simulink model "starshotsimv5"  (R2021a)
settings: Solver=VariableStepAuto  StartTime=0.0  StopTime=6000  FixedStep=0.01  MaxStep=4.0  MinStep=.001  RelTol=1e-6
values from neighbouring files (symbols this model uses):
  B0 = 3.12e-5    (= 3.12e-05)    [starshot_ACS_setup.m]
  dT = 0.01    [scr_EKF.m]    (also in starshot_ACS_setup.m = 0.1)
  G = 6.67e-11    [starshot_ACS_setup.m]
  Hd = H    [scr_EKF.m]    (also in starshot_ACS_setup.m)
  k_noise = 1    [scr_EKF.m]    (also in starshot_ACS_setup.m = 3e-05)
  M_Earth = 5.972e24    (= 5.972e+24)    [starshot_ACS_setup.m]
  Q = [100,  0,  0 ... (first row only)    [scr_EKF.m]    (also in starshot_ACS_setup.m = 0.02*diag([0.008,0.07,0.005,0.1,0.1,0.1]))
  q0 = [qmatlab(2:4),qmatlab(1)]'    [starshot_ACS_setup.m]
  R_Earth = 6.378e6    (= 6378000)    [starshot_ACS_setup.m]
  Rd = (1/dT)*R    [scr_EKF.m]    (also in starshot_ACS_setup.m = Rn)
  Rn = [[ 2.02559220e-01,  5.17515015e-03, -3.16669361e-02, -1.76503506e-04, -3.74891174e-05, -7.75657503e-05] ... (first row only)    [starshot_ACS_setup.m]
undefined symbols (not defined in the file or in its folder): DiscIntNeverNeededParam, starshot
libraries: vrlib x2, simulink x2, dspmathops x1
settings Model: Creator=armen  LastModifiedBy=soumy
settings DataIOCC: SaveFormat=Array  ReturnWorkspaceOutputs=off
settings OptimizationCC: DefaultParameterBehavior=Inlined  UseDivisionForNetSlopeComputation=on  UseFloatMulNetSlope=on  InlineInvariantSignals=on  PassReuseOutputArgsAs=Individual arguments  ZeroExternalMemoryAtStartup=off  ZeroInternalMemoryAtStartup=off  NoFixptDivByZeroProtection=on  EfficientFloat2IntCast=on  LifeSpan=1  EfficientTunableParamExpr=on
settings DebuggingCC: ParameterTunabilityLossMsg=error  SFMachineParentedDataDiag=warning  ArithmeticOperatorsInVariantConditions=warning
settings HardwareCC: ProdBitPerPointer=32  ProdBitPerSizeT=32  ProdBitPerPtrDiffT=32  ProdLargestAtomicInteger=Long  ProdLargestAtomicFloat=Double  ProdWordSize=32  ProdHWDeviceType=ARM Compatible->ARM Cortex
settings SFSimCC: SimUseLocalCustomCode=off  MATLABDynamicMemAlloc=off  CustomCodeUndefinedFunction=UseInterfaceOnly  SimTargetLang=C++
settings RTWCC: SystemTargetFile=ert.tlc  GenCodeOnly=on  TemplateMakefile=ert_default_tmf  GenerateReport=on  RTWUseLocalCustomCode=off  IncludeHyperlinkInReport=on  LaunchReport=on  TargetLang=C++  GenerateTraceInfo=on  GenerateTraceReport=on  GenerateTraceReportSl=on  GenerateTraceReportSf=on  GenerateTraceReportEml=on
settings CodeAppCC: ForceParamTrailComments=on  IgnoreCustomStorageClasses=off  OperatorAnnotations=on  SimulinkDataObjDesc=on  SFDataObjDesc=on  MATLABFcnDesc=on  CustomSymbolStrGlobalVar=rt$N$M  CustomSymbolStrType=$N$M  CustomSymbolStrFcn=$N$M$F  CustomSymbolStrMacro=$N$M  InsertBlockDesc=on  StateflowObjectComments=on  MATLABSourceComments=on
settings ERTTargetCC: TargetLangStandard=C++03 (ISO)  GenerateSampleERTMain=on  IncludeMdlTerminateFcn=off  CombineSignalStateStructs=on  SupportAbsoluteTime=off  CodeInterfacePackaging=C++ class  SupportComplex=off  SupportNonInlinedSFcns=on  InlinedParameterPlacement=NonHierarchical  RootIOFormat=Structure reference  ERTCustomFileTemplate=example_file_process.tlc  ERTFilePackagingFormat=CompactWithDataFile

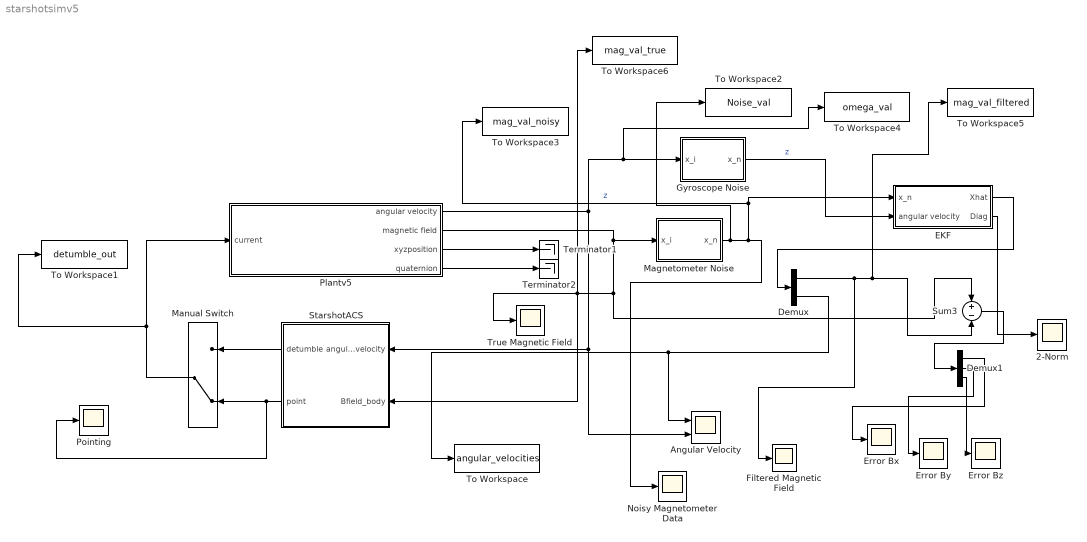
== system starshotsimv5 ==
  2-Norm : Scope
  Angular Velocity : Scope  NumInputPorts=2
  Demux : Demux  Outputs=2
  Demux1 : Demux  Outputs=3
  EKF : Subsystem  TreatAsAtomicUnit=on
      settings: MinAlgLoopOccurrences=on
  Error Bx : Scope
  Error By : Scope
  Error Bz : Scope
  Filtered Magnetic Field : Scope
  Gyroscope Noise : Subsystem
  Magnetometer Noise : Subsystem  TreatAsAtomicUnit=on
      settings: MinAlgLoopOccurrences=on
  Manual Switch : ManualSwitch  CurrentSetting=0
  Noisy Magnetometer Data : Scope
  Plantv5 : Subsystem  TreatAsAtomicUnit=on
  Pointing : Scope
  StarshotACS : Subsystem  TreatAsAtomicUnit=on
  Sum3 : Sum  Inputs=+-
  Terminator1 : Terminator
  Terminator2 : Terminator
  To Workspace : ToWorkspace  VariableName=angular_velocities  SaveFormat=Timeseries  SampleTime=-1
  To Workspace1 : ToWorkspace  VariableName=detumble_out  SaveFormat=Timeseries  SampleTime=-1
  To Workspace2 : ToWorkspace  VariableName=Noise_val  SaveFormat=Timeseries  SampleTime=-1
  To Workspace3 : ToWorkspace  VariableName=mag_val_noisy  SaveFormat=Timeseries  SampleTime=-1
  To Workspace4 : ToWorkspace  VariableName=omega_val  SaveFormat=Timeseries  SampleTime=-1
  To Workspace5 : ToWorkspace  VariableName=mag_val_filtered  SaveFormat=Timeseries  SampleTime=-1
  To Workspace6 : ToWorkspace  VariableName=mag_val_true  SaveFormat=Timeseries  SampleTime=-1
  True Magnetic Field : Scope
  wires:
  Plantv5/2(magnetic field) -> Sum3/1, StarshotACS/2(Bfield_body), To Workspace6/1, True Magnetic Field/1, Magnetometer Noise/1(x_i)
  Plantv5/1(angular velocity) -> To Workspace4/1, Gyroscope Noise/1(x_i), Angular Velocity/2, StarshotACS/1(angularvelocity)
  Plantv5/3(xyzposition) -> Terminator1/1
  Plantv5/4(quaternion) -> Terminator2/1
  StarshotACS/2(point) -> Pointing/1, Manual Switch/2
  StarshotACS/1(detumble) -> Manual Switch/1
  Manual Switch/1 -> To Workspace1/1, Plantv5/1(current)
  Magnetometer Noise/1(x_n) -> To Workspace2/1, To Workspace3/1, EKF/1(x_n), Noisy Magnetometer Data/1  "z"
  EKF/1(Xhat) -> Demux/1
  Demux/1 -> To Workspace5/1, Sum3/2, Filtered Magnetic Field/1
  Demux/2 -> To Workspace/1, Angular Velocity/1
  Gyroscope Noise/1(x_n) -> EKF/2(angular velocity)  "z"
  Sum3/1 -> Demux1/1
  Demux1/1 -> Error Bx/1
  Demux1/2 -> Error By/1
  Demux1/3 -> Error Bz/1
  EKF/2(Diag) -> 2-Norm/1

== system starshotsimv5/EKF ==
  x_n : Inport
  angular velocity : Inport  Port=2
  EKF_Primary : Subsystem
  Jacobian : MATLAB Function  TreatAsAtomicUnit=on
  Scope : Scope  NumInputPorts=2
  Vector Concatenate : Concatenate
  Xhat : Outport
  Diag : Outport  Port=2
  wires:
  EKF_Primary/2(sqrtPii) -> Diag/1
  Jacobian/1(J) -> EKF_Primary/2(J)
  EKF_Primary/1(Xhat) -> Scope/2, Xhat/1
  angular velocity/1 -> Vector Concatenate/2, Jacobian/2(angular_velocities)
  x_n/1 -> Vector Concatenate/1, Jacobian/1(B_body)  "z"
  Vector Concatenate/1 -> Scope/1, EKF_Primary/1(Z)

== system starshotsimv5/Gyroscope Noise ==
  x_i : Inport
  From Workspace : FromWorkspace  VariableName=w_noise
  Gain2 : Gain  Gain=k_noise
  Sum2 : Sum  Inputs=++|
  x_n : Outport  VectorParamsAs1DForOutWhenUnconnected=off
  wires:
  From Workspace/1 -> Gain2/1
  Gain2/1 -> Sum2/1
  x_i/1 -> Sum2/2
  Sum2/1 -> x_n/1

== system starshotsimv5/Magnetometer Noise ==
  x_i : Inport
  Demux : Demux  Outputs=3
  From Workspace : FromWorkspace  VariableName=mag_noise
  Gain2 : Gain  Gain=k_noise
  Random Number : RandomNumber  Mean=1  Seed=[1 2 3]  SampleTime=0.1
  Scope : Scope
  Sum2 : Sum  Inputs=++|
  To Workspace : ToWorkspace  VariableName=noise_x  SaveFormat=Timeseries  SampleTime=-1
  x_n : Outport  VectorParamsAs1DForOutWhenUnconnected=off
  wires:
  Gain2/1 -> Demux/1, Sum2/1
  x_i/1 -> Sum2/2
  Sum2/1 -> x_n/1
  Demux/1 -> To Workspace/1, Scope/1
  From Workspace/1 -> Gain2/1

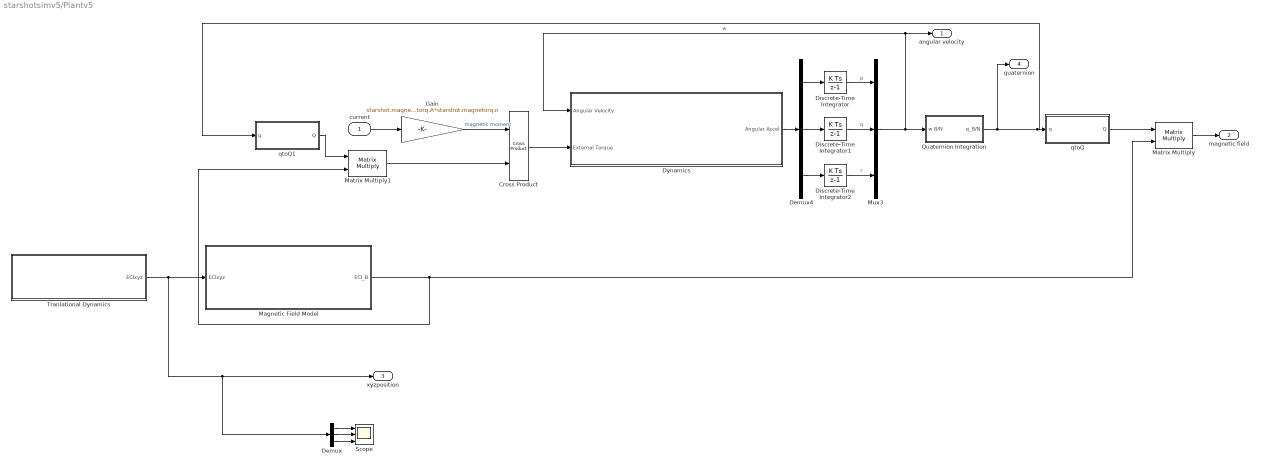
== system starshotsimv5/Plantv5 ==
  current : Inport
  Cross Product : vrlib/Utilities/Cross Product
  Demux : Demux  Outputs=3
  Demux4 : Demux  Outputs=3
  Discrete-Time Integrator : DiscreteIntegrator  InitialCondition=starshot.IC.w(1)  SampleTime=-1  ICPrevOutput=DiscIntNeverNeededParam  ICPrevScaledInput=DiscIntNeverNeededParam
  Discrete-Time Integrator1 : DiscreteIntegrator  InitialCondition=starshot.IC.w(2)  SampleTime=-1  ICPrevOutput=DiscIntNeverNeededParam  ICPrevScaledInput=DiscIntNeverNeededParam
  Discrete-Time Integrator2 : DiscreteIntegrator  InitialCondition=starshot.IC.w(3)  SampleTime=-1  ICPrevOutput=DiscIntNeverNeededParam  ICPrevScaledInput=DiscIntNeverNeededParam
  Dynamics : Subsystem  TreatAsAtomicUnit=on
  Gain : Gain  Gain=starshot.magnetorq.A*starshot.magnetorq.n
  Magnetic Field Model : Subsystem  TreatAsAtomicUnit=on
  Matrix Multiply : Product  Multiplication=Matrix(*)
  Matrix Multiply1 : Product  Multiplication=Matrix(*)
  Mux3 : Mux  Inputs=3
  Quaternion Integration : Subsystem
  Scope : Scope  NumInputPorts=3
  Tranlational Dynamics : Subsystem  TreatAsAtomicUnit=on
  qtoQ : Subsystem  TreatAsAtomicUnit=on
  qtoQ1 : Subsystem  TreatAsAtomicUnit=on
  angular velocity : Outport
  magnetic field : Outport  Port=2
  xyzposition : Outport  Port=3
  quaternion : Outport  Port=4
  wires:
  Matrix Multiply/1 -> magnetic field/1
  Magnetic Field Model/1(ECI_B) -> Matrix Multiply1/2, Matrix Multiply/2
  Discrete-Time Integrator1/1 -> Mux3/2  "q"
  Discrete-Time Integrator2/1 -> Mux3/3  "r"
  Demux4/3 -> Discrete-Time Integrator2/1
  Demux4/1 -> Discrete-Time Integrator/1
  Tranlational Dynamics/1(ECIxyz) -> Demux/1, xyzposition/1, Magnetic Field Model/1(ECIxyz)
  Quaternion Integration/1(q_B/N) -> qtoQ1/1(q), qtoQ/1(q), quaternion/1
  Dynamics/1(Angular Accel) -> Demux4/1
  Mux3/1 -> Quaternion Integration/1(w B/N), Dynamics/1(Angular Velocity), angular velocity/1  "w"
  current/1 -> Gain/1
  Gain/1 -> Cross Product/1  "magnetic moment"
  Discrete-Time Integrator/1 -> Mux3/1  "p"
  Demux4/2 -> Discrete-Time Integrator1/1
  Demux/2 -> Scope/2
  Demux/1 -> Scope/1
  Demux/3 -> Scope/3
  qtoQ/1(Q) -> Matrix Multiply/1
  Matrix Multiply1/1 -> Cross Product/2
  qtoQ1/1(Q) -> Matrix Multiply1/1
  Cross Product/1 -> Dynamics/2(External Torque)

== system starshotsimv5/StarshotACS ==
  angularvelocity : Inport
  Bfield_body : Inport  Port=2
  KD_controller : Subsystem
  Orientation controller : Subsystem
  detumble : Outport
  point : Outport  Port=2
  wires:
  KD_controller/1(Dipole) -> detumble/1
  Orientation controller/1(Dipole) -> point/1
  Bfield_body/1 -> KD_controller/2(B(body)), Orientation controller/2(B(body))  "Bfield_body"
  angularvelocity/1 -> Orientation controller/1(Omega), KD_controller/1(Omega)  "angularvelocity"

== system starshotsimv5/EKF/EKF_Primary ==
  Z : Inport
  J : Inport  Port=2
  Kalman corrector : MATLAB Function  TreatAsAtomicUnit=on
  Kalman predictor : MATLAB Function  TreatAsAtomicUnit=on
  To Workspace : ToWorkspace  VariableName=Z_data  SaveFormat=Timeseries  SampleTime=-1
  Unit Delay - P : UnitDelay  InitialCondition=Rn  SampleTime=-1  HasFrameUpgradeWarning=on
  Unit Delay - X : UnitDelay  InitialCondition=[3.42e-05,-3.0e-06,-9.28e-05,0.06, -0.05, 0.07]'  SampleTime=-1  HasFrameUpgradeWarning=on
  sqrt(Pii) : MATLAB Function  TreatAsAtomicUnit=on
  Xhat : Outport  PortDimensions=6
  sqrtPii : Outport  Port=2  VectorParamsAs1DForOutWhenUnconnected=off
  wires:
  Unit Delay - P/1 -> Kalman predictor/3(P_k_k)
  J/1 -> Kalman predictor/1(J_k_k)
  Kalman corrector/2(P_k1_k1) -> sqrt(Pii)/1(u), Unit Delay - P/1
  Kalman corrector/1(X_k1_k1) -> Xhat/1, Unit Delay - X/1
  sqrt(Pii)/1(y) -> sqrtPii/1
  Kalman predictor/1(X_k1_k) -> Kalman corrector/2(X_k1_k)
  Kalman predictor/2(P_k1_k) -> Kalman corrector/3(P_k1_k)
  Unit Delay - X/1 -> Kalman predictor/2(X_k_k)
  Z/1 -> To Workspace/1, Kalman corrector/1(Z)

== system starshotsimv5/Plantv5/Dynamics ==
  Angular Velocity : Inport
  External Torque : Inport  Port=2
  Constant : Constant  Value=starshot.IC.massproperties.I
  Constant1 : Constant  Value=starshot.IC.massproperties.Iinv
  Cross Product : vrlib/Utilities/Cross Product
  Product : Product  Multiplication=Matrix(*)
  Product1 : Product  Multiplication=Matrix(*)
  Sum : Sum  Inputs=+-
  Angular Accel : Outport
  wires:
  Angular Velocity/1 -> Cross Product/1, Product/2
  Constant/1 -> Product/1
  Product/1 -> Cross Product/2
  External Torque/1 -> Sum/1
  Constant1/1 -> Product1/1
  Product1/1 -> Angular Accel/1
  Sum/1 -> Product1/2
  Cross Product/1 -> Sum/2

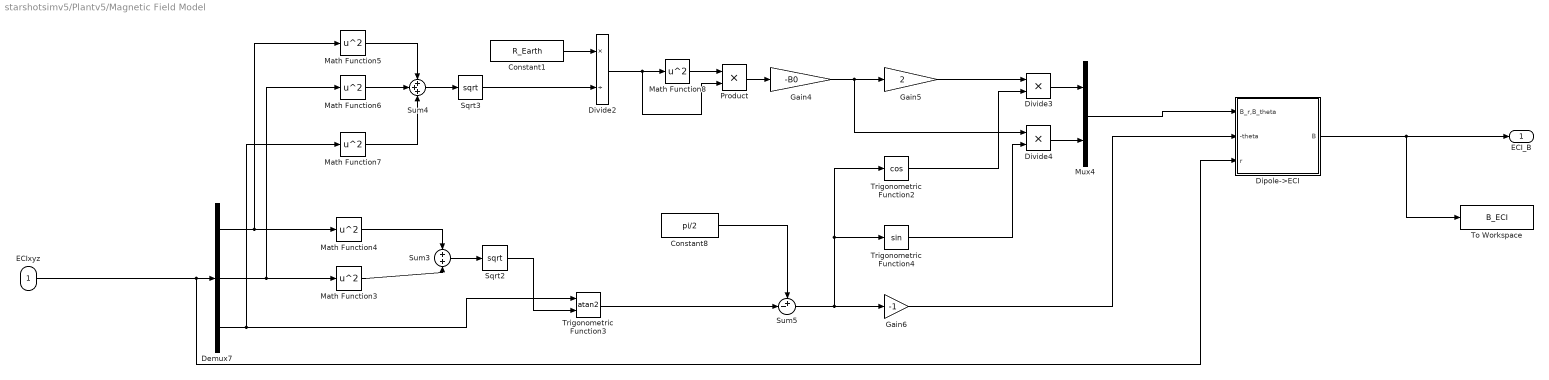
== system starshotsimv5/Plantv5/Magnetic Field Model ==
  ECIxyz : Inport
  Constant1 : Constant  Value=R_Earth
  Constant8 : Constant  Value=pi/2
  Demux7 : Demux  Outputs=3
  Dipole->ECI : Subsystem  TreatAsAtomicUnit=on
  Divide2 : Product  Inputs=*/
  Divide3 : Product  Inputs=**
  Divide4 : Product  Inputs=**
  Gain4 : Gain  Gain=-B0
  Gain5 : Gain  Gain=2
  Gain6 : Gain  Gain=-1
  Math Function{3..8} (6 alike) : Math  Operator=square  SignedPower=on  SaturateOnIntegerOverflow=on
  Mux4 : Mux  Inputs=2
  Product : Product
  Sqrt2 : Sqrt  SaturateOnIntegerOverflow=on
  Sqrt3 : Sqrt  SaturateOnIntegerOverflow=on
  Sum3 : Sum
  Sum4 : Sum  Inputs=+++
  Sum5 : Sum  Inputs=+-|
  To Workspace : ToWorkspace  VariableName=B_ECI  SaveFormat=Timeseries  SampleTime=-1
  Trigonometric Function2 : Trigonometry  Operator=cos
  Trigonometric Function3 : Trigonometry  Operator=atan2
  Trigonometric Function4 : Trigonometry
  ECI_B : Outport
  wires:
  Math Function7/1 -> Sum4/3
  Constant1/1 -> Divide2/1
  Math Function5/1 -> Sum4/1
  Math Function4/1 -> Sum3/1
  Demux7/3 -> Math Function7/1, Trigonometric Function3/1
  Sqrt2/1 -> Trigonometric Function3/2
  Product/1 -> Gain4/1
  Math Function8/1 -> Product/1
  Gain5/1 -> Divide3/1
  Sqrt3/1 -> Divide2/2
  Sum4/1 -> Sqrt3/1
  Divide2/1 -> Product/2, Math Function8/1
  Sum3/1 -> Sqrt2/1
  Math Function3/1 -> Sum3/2
  Demux7/1 -> Math Function5/1, Math Function4/1
  Gain4/1 -> Gain5/1, Divide4/1
  Trigonometric Function2/1 -> Divide3/2
  Math Function6/1 -> Sum4/2
  Demux7/2 -> Math Function6/1, Math Function3/1
  Sum5/1 -> Trigonometric Function2/1, Trigonometric Function4/1, Gain6/1
  Trigonometric Function4/1 -> Divide4/2
  Gain6/1 -> Dipole->ECI/2(-theta)
  Divide4/1 -> Mux4/2
  Trigonometric Function3/1 -> Sum5/2
  Constant8/1 -> Sum5/1
  Mux4/1 -> Dipole->ECI/1(B_r,B_theta)
  Divide3/1 -> Mux4/1
  ECIxyz/1 -> Dipole->ECI/3(r), Demux7/1
  Dipole->ECI/1(B) -> To Workspace/1, ECI_B/1

== system starshotsimv5/Plantv5/Quaternion Integration ==
  w B/N : Inport
  Discrete-Time Integrator1 : DiscreteIntegrator  InitialCondition=q0  SampleTime=-1  ICPrevOutput=DiscIntNeverNeededParam  ICPrevScaledInput=DiscIntNeverNeededParam
  q_normalize : Subsystem
  qderiv : Subsystem
  q_B/N : Outport
  wires:
  w B/N/1 -> qderiv/1(w)
  q_normalize/1(q_out) -> qderiv/2(q), q_B/N/1
  Discrete-Time Integrator1/1 -> q_normalize/1(q_in)
  qderiv/1(qd) -> Discrete-Time Integrator1/1

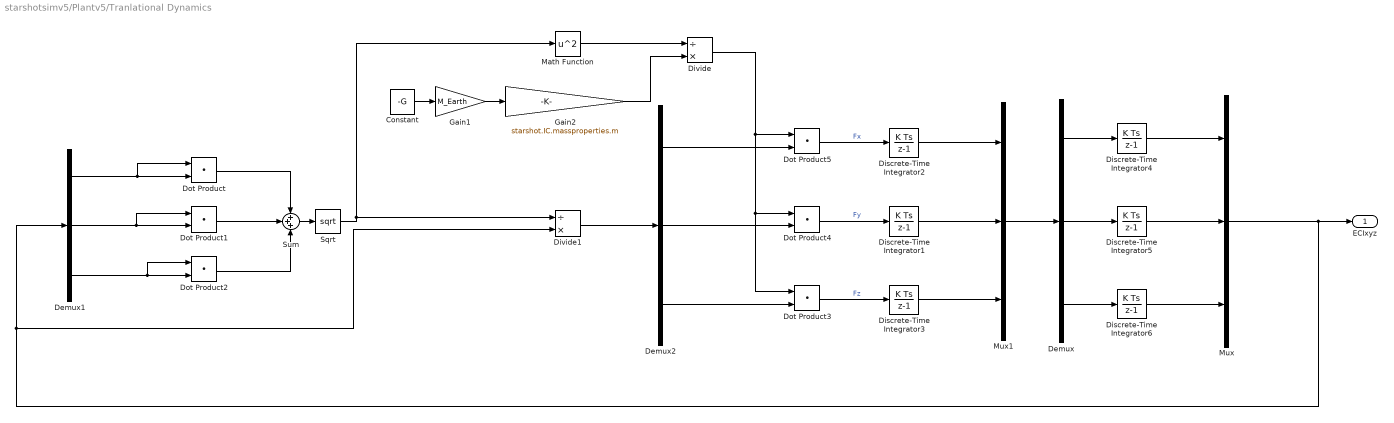
== system starshotsimv5/Plantv5/Tranlational Dynamics ==
  Constant : Constant  Value=-G
  Demux : Demux  Outputs=3
  Demux1 : Demux  Outputs=3
  Demux2 : Demux  Outputs=3
  Discrete-Time Integrator1 : DiscreteIntegrator  InitialCondition=starshot.IC.ydot  SampleTime=-1  ICPrevOutput=DiscIntNeverNeededParam  ICPrevScaledInput=DiscIntNeverNeededParam
  Discrete-Time Integrator2 : DiscreteIntegrator  InitialCondition=starshot.IC.xdot  SampleTime=-1  ICPrevOutput=DiscIntNeverNeededParam  ICPrevScaledInput=DiscIntNeverNeededParam
  Discrete-Time Integrator3 : DiscreteIntegrator  InitialCondition=starshot.IC.zdot  SampleTime=-1  ICPrevOutput=DiscIntNeverNeededParam  ICPrevScaledInput=DiscIntNeverNeededParam
  Discrete-Time Integrator4 : DiscreteIntegrator  InitialCondition=starshot.IC.x  SampleTime=-1  ICPrevOutput=DiscIntNeverNeededParam  ICPrevScaledInput=DiscIntNeverNeededParam
  Discrete-Time Integrator5 : DiscreteIntegrator  InitialCondition=starshot.IC.y  SampleTime=-1  ICPrevOutput=DiscIntNeverNeededParam  ICPrevScaledInput=DiscIntNeverNeededParam
  Discrete-Time Integrator6 : DiscreteIntegrator  InitialCondition=starshot.IC.z  SampleTime=-1  ICPrevOutput=DiscIntNeverNeededParam  ICPrevScaledInput=DiscIntNeverNeededParam
  Divide : Product  Inputs=/*
  Divide1 : Product  Inputs=/*
  Dot Product{,1..5} (6 alike) : DotProduct  InputSameDT=on  OutDataTypeStr=Inherit: Inherit via internal rule
  Gain1 : Gain  Gain=M_Earth
  Gain2 : Gain  Gain=starshot.IC.massproperties.m
  Math Function : Math  Operator=square  SignedPower=on  SaturateOnIntegerOverflow=on
  Mux : Mux  Inputs=3
  Mux1 : Mux  Inputs=3
  Sqrt : Sqrt  SaturateOnIntegerOverflow=on
  Sum : Sum  Inputs=+++
  ECIxyz : Outport
  wires:
  Discrete-Time Integrator6/1 -> Mux/3
  Discrete-Time Integrator5/1 -> Mux/2
  Discrete-Time Integrator4/1 -> Mux/1
  Demux/3 -> Discrete-Time Integrator6/1
  Demux/1 -> Discrete-Time Integrator4/1
  Mux1/1 -> Demux/1
  Discrete-Time Integrator3/1 -> Mux1/3
  Demux/2 -> Discrete-Time Integrator5/1
  Demux1/2 -> Dot Product1/1, Dot Product1/2
  Sum/1 -> Sqrt/1
  Dot Product4/1 -> Discrete-Time Integrator1/1  "Fy"
  Demux1/1 -> Dot Product/1, Dot Product/2
  Dot Product3/1 -> Discrete-Time Integrator3/1  "Fz"
  Divide/1 -> Dot Product3/1, Dot Product4/1, Dot Product5/1
  Dot Product1/1 -> Sum/2
  Demux1/3 -> Dot Product2/1, Dot Product2/2
  Dot Product2/1 -> Sum/3
  Demux2/2 -> Dot Product4/2
  Demux2/3 -> Dot Product3/2
  Math Function/1 -> Divide/1
  Discrete-Time Integrator1/1 -> Mux1/2
  Gain1/1 -> Gain2/1
  Demux2/1 -> Dot Product5/2
  Dot Product5/1 -> Discrete-Time Integrator2/1  "Fx"
  Dot Product/1 -> Sum/1
  Constant/1 -> Gain1/1
  Divide1/1 -> Demux2/1
  Gain2/1 -> Divide/2
  Sqrt/1 -> Math Function/1, Divide1/1
  Discrete-Time Integrator2/1 -> Mux1/1
  Mux/1 -> ECIxyz/1, Divide1/2, Demux1/1

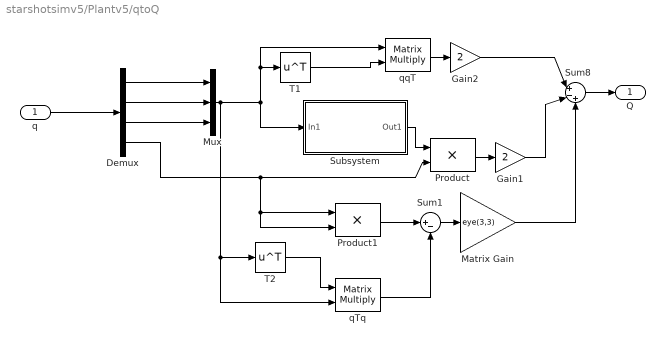
== system starshotsimv5/Plantv5/qtoQ ==
  q : Inport
  Demux : Demux
      settings: DisplayOption=none
  Gain1 : Gain  Gain=2  SaturateOnIntegerOverflow=on  OutDataTypeStr=Inherit: Same as input  ParamDataTypeStr=Inherit: Same as input
  Gain2 : Gain  Gain=2  SaturateOnIntegerOverflow=on  OutDataTypeStr=Inherit: Same as input  ParamDataTypeStr=Inherit: Same as input
  Matrix Gain : Gain  Gain=eye(3,3)  SaturateOnIntegerOverflow=on  OutDataTypeStr=Inherit: Same as input  ParamDataTypeStr=Inherit: Same as input
  Mux : Mux  Inputs=3
  Product : Product  InputSameDT=on  SaturateOnIntegerOverflow=on  OutDataTypeStr=Inherit: Same as first input
  Product1 : Product  InputSameDT=on  SaturateOnIntegerOverflow=on  OutDataTypeStr=Inherit: Same as first input
  Subsystem : Subsystem
      mask Display: disp('3x3 cross matrix')
  Sum1 : Sum  Inputs=|+-  InputSameDT=on  SaturateOnIntegerOverflow=on  OutDataTypeStr=Inherit: Same as first input
  Sum8 : Sum  Inputs=|+-+  InputSameDT=on  SaturateOnIntegerOverflow=on  OutDataTypeStr=Inherit: Same as first input
  T1 : Math  Operator=transpose  SignedPower=on  SaturateOnIntegerOverflow=on
  T2 : Math  Operator=transpose  SignedPower=on  SaturateOnIntegerOverflow=on
  qTq : Product  Multiplication=Matrix(*)  InputSameDT=on  SaturateOnIntegerOverflow=on  OutDataTypeStr=Inherit: Same as first input
  qqT : Product  Multiplication=Matrix(*)  InputSameDT=on  SaturateOnIntegerOverflow=on  OutDataTypeStr=Inherit: Same as first input
  Q : Outport
  wires:
  q/1 -> Demux/1
  Demux/1 -> Mux/1
  Matrix Gain/1 -> Sum8/3
  Demux/2 -> Mux/2
  Demux/3 -> Mux/3
  T2/1 -> qTq/1
  Demux/4 -> Product1/2, Product1/1, Product/2
  Product/1 -> Gain1/1
  qqT/1 -> Gain2/1
  Mux/1 -> qTq/2, T2/1, qqT/1, T1/1, Subsystem/1(In1)
  Sum8/1 -> Q/1
  Subsystem/1(Out1) -> Product/1
  Product1/1 -> Sum1/1
  Gain2/1 -> Sum8/1
  T1/1 -> qqT/2
  Gain1/1 -> Sum8/2
  qTq/1 -> Sum1/2
  Sum1/1 -> Matrix Gain/1

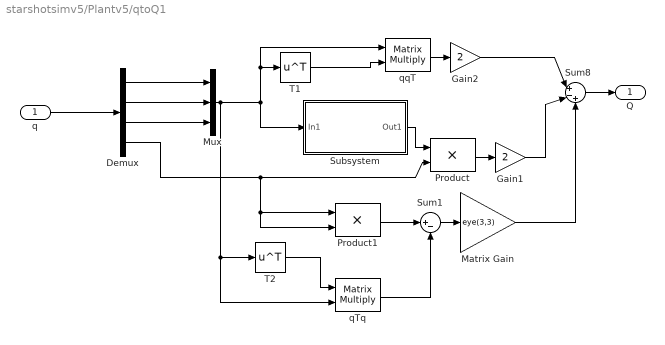
== system starshotsimv5/Plantv5/qtoQ1 ==
  q : Inport
  Demux : Demux
      settings: DisplayOption=none
  Gain1 : Gain  Gain=2  SaturateOnIntegerOverflow=on  OutDataTypeStr=Inherit: Same as input  ParamDataTypeStr=Inherit: Same as input
  Gain2 : Gain  Gain=2  SaturateOnIntegerOverflow=on  OutDataTypeStr=Inherit: Same as input  ParamDataTypeStr=Inherit: Same as input
  Matrix Gain : Gain  Gain=eye(3,3)  SaturateOnIntegerOverflow=on  OutDataTypeStr=Inherit: Same as input  ParamDataTypeStr=Inherit: Same as input
  Mux : Mux  Inputs=3
  Product : Product  InputSameDT=on  SaturateOnIntegerOverflow=on  OutDataTypeStr=Inherit: Same as first input
  Product1 : Product  InputSameDT=on  SaturateOnIntegerOverflow=on  OutDataTypeStr=Inherit: Same as first input
  Subsystem : Subsystem
      mask Display: disp('3x3 cross matrix')
  Sum1 : Sum  Inputs=|+-  InputSameDT=on  SaturateOnIntegerOverflow=on  OutDataTypeStr=Inherit: Same as first input
  Sum8 : Sum  Inputs=|+-+  InputSameDT=on  SaturateOnIntegerOverflow=on  OutDataTypeStr=Inherit: Same as first input
  T1 : Math  Operator=transpose  SignedPower=on  SaturateOnIntegerOverflow=on
  T2 : Math  Operator=transpose  SignedPower=on  SaturateOnIntegerOverflow=on
  qTq : Product  Multiplication=Matrix(*)  InputSameDT=on  SaturateOnIntegerOverflow=on  OutDataTypeStr=Inherit: Same as first input
  qqT : Product  Multiplication=Matrix(*)  InputSameDT=on  SaturateOnIntegerOverflow=on  OutDataTypeStr=Inherit: Same as first input
  Q : Outport
  wires:
  Sum1/1 -> Matrix Gain/1
  qTq/1 -> Sum1/2
  Gain1/1 -> Sum8/2
  T1/1 -> qqT/2
  Gain2/1 -> Sum8/1
  Product1/1 -> Sum1/1
  Subsystem/1(Out1) -> Product/1
  Sum8/1 -> Q/1
  Mux/1 -> Subsystem/1(In1), T1/1, qqT/1, T2/1, qTq/2
  qqT/1 -> Gain2/1
  Product/1 -> Gain1/1
  Demux/4 -> Product/2, Product1/1, Product1/2
  T2/1 -> qTq/1
  Demux/3 -> Mux/3
  Demux/2 -> Mux/2
  Matrix Gain/1 -> Sum8/3
  Demux/1 -> Mux/1
  q/1 -> Demux/1

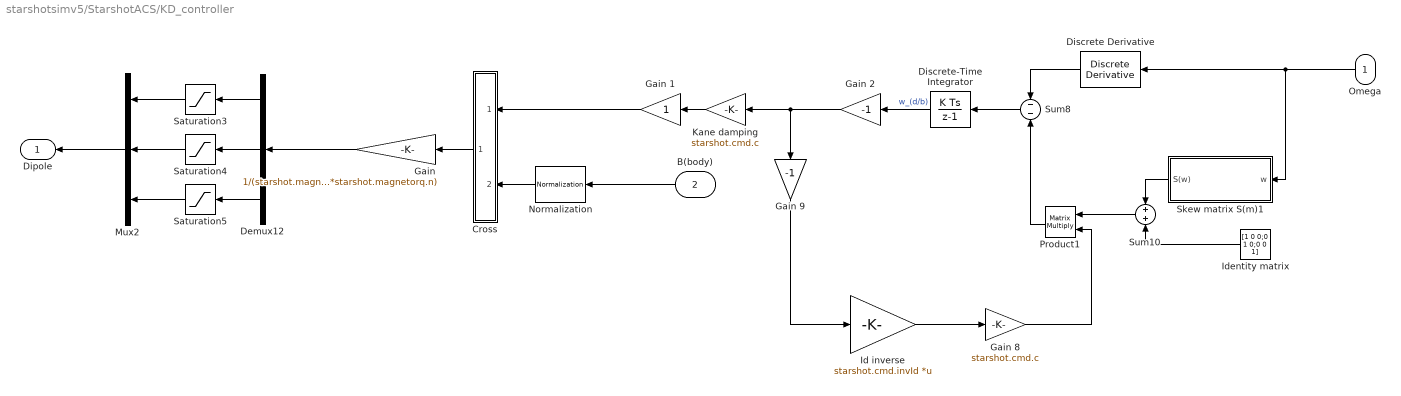
== system starshotsimv5/StarshotACS/KD_controller ==
  Omega : Inport
  B(body) : Inport  Port=2
  Cross : Subsystem
  Demux12 : Demux  Outputs=3
  Discrete Derivative : simulink/Discrete/Discrete Derivative  gainval=1.0  ICPrevScaledInput=0.0  OutMin=[]  OutMax=[]  OutDataType=fixdt(1, 16)  OutScaling=2^-10  DoSatur=off
  Discrete-Time Integrator : DiscreteIntegrator  InitialCondition=starshot.cmd.wdb0  SampleTime=-1  ICPrevOutput=DiscIntNeverNeededParam  ICPrevScaledInput=DiscIntNeverNeededParam
  Gain : Gain  Gain=1/(starshot.magnetorq.A*starshot.magnetorq.n)
  Gain 1 : Gain  SaturateOnIntegerOverflow=on  OutDataTypeStr=Inherit: Same as input  ParamDataTypeStr=Inherit: Same as input
  Gain 2 : Gain  Gain=-1  SaturateOnIntegerOverflow=on  OutDataTypeStr=Inherit: Same as input  ParamDataTypeStr=Inherit: Same as input
  Gain 8 : Gain  Gain=starshot.cmd.c  SaturateOnIntegerOverflow=on  OutDataTypeStr=Inherit: Same as input  ParamDataTypeStr=Inherit: Same as input
  Gain 9 : Gain  Gain=-1  SaturateOnIntegerOverflow=on  OutDataTypeStr=Inherit: Same as input  ParamDataTypeStr=Inherit: Same as input
  Id inverse : Gain  Gain=starshot.cmd.invId  Multiplication=Matrix(K*u)  SaturateOnIntegerOverflow=on  OutDataTypeStr=Inherit: Same as input  ParamDataTypeStr=Inherit: Same as input
  Identity matrix : Constant  Value=[1 0 0;0 1 0;0 0 1]
  Kane damping : Gain  Gain=starshot.cmd.c  SaturateOnIntegerOverflow=on  OutDataTypeStr=Inherit: Same as input  ParamDataTypeStr=Inherit: Same as input
  Mux2 : Mux  Inputs=3
  Normalization : dspmathops/Normalization  NormType=Squared 2-norm  Bias=1e-10  NormOver=Each column  Dimension=1  roundingMode=Floor  overflowMode=off  accumDataTypeStr=Inherit: Same as product output  accumLastDataTypeStr=Inherit: Same as product output  outputDataTypeStr=Inherit: Same as product output  outputMin=[]  outputMax=[]  outputLastDataTypeStr=Inherit: Same as product output
  Product1 : Product  Multiplication=Matrix(*)
  Saturation3 : Saturate  UpperLimit=starshot.magnetorq.m_max_x/(starshot.magnetorq.A*starshot.magnetorq.n)  LowerLimit=-starshot.magnetorq.m_max_x/(starshot.magnetorq.A*starshot.magnetorq.n)
  Saturation4 : Saturate  UpperLimit=starshot.magnetorq.m_max_y/(starshot.magnetorq.A*starshot.magnetorq.n)  LowerLimit=-starshot.magnetorq.m_max_y/(starshot.magnetorq.A*starshot.magnetorq.n)
  Saturation5 : Saturate  UpperLimit=starshot.magnetorq.m_max_z/(starshot.magnetorq.A*starshot.magnetorq.n)  LowerLimit=-starshot.magnetorq.m_max_z/(starshot.magnetorq.A*starshot.magnetorq.n)
  Skew matrix S(m)1 : Subsystem
  Sum10 : Sum  Inputs=+|+  InputSameDT=on  SaturateOnIntegerOverflow=on  OutDataTypeStr=Inherit: Same as first input
  Sum8 : Sum  Inputs=--
  Dipole : Outport
  wires:
  Discrete-Time Integrator/1 -> Gain 2/1  "w_(d/b)"
  Omega/1 -> Discrete Derivative/1, Skew matrix S(m)1/1(w)
  B(body)/1 -> Normalization/1
  Cross/1(AxB) -> Gain/1
  Gain 2/1 -> Kane damping/1, Gain 9/1
  Normalization/1 -> Cross/2(B)
  Kane damping/1 -> Gain 1/1
  Discrete Derivative/1 -> Sum8/1
  Sum8/1 -> Discrete-Time Integrator/1
  Gain 8/1 -> Product1/2
  Id inverse/1 -> Gain 8/1
  Skew matrix S(m)1/1(S(w)) -> Sum10/1
  Identity matrix/1 -> Sum10/2
  Gain 9/1 -> Id inverse/1
  Sum10/1 -> Product1/1
  Product1/1 -> Sum8/2
  Gain 1/1 -> Cross/1(A)
  Gain/1 -> Demux12/1
  Demux12/1 -> Saturation3/1
  Saturation3/1 -> Mux2/1
  Saturation5/1 -> Mux2/3
  Demux12/2 -> Saturation4/1
  Saturation4/1 -> Mux2/2
  Demux12/3 -> Saturation5/1
  Mux2/1 -> Dipole/1

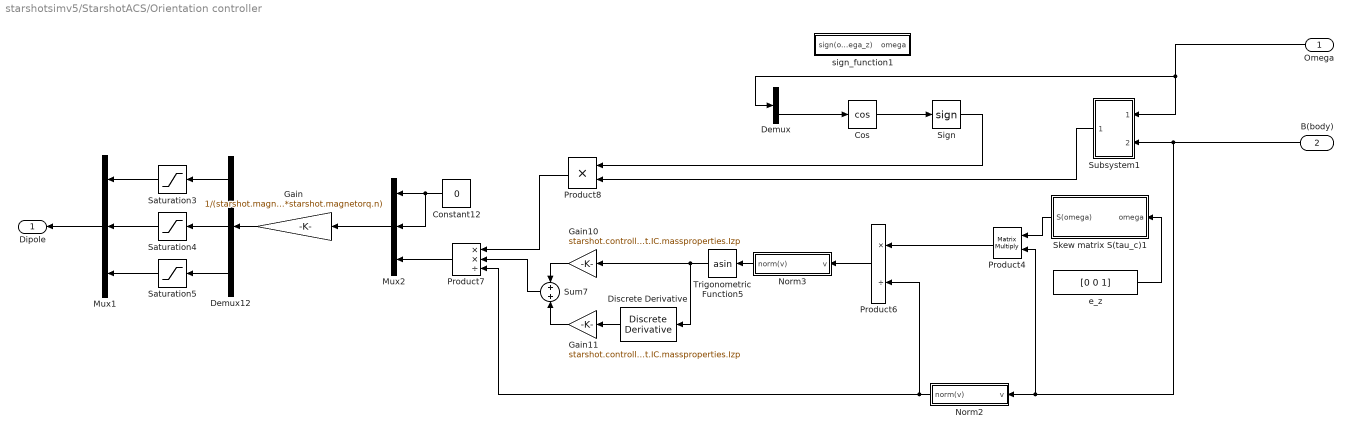
== system starshotsimv5/StarshotACS/Orientation controller ==
  Omega : Inport
  B(body) : Inport  Port=2
  Constant12 : Constant  Value=0
  Cos : Trigonometry  Operator=cos
  Demux : Demux  Outputs=3
  Demux12 : Demux  Outputs=3
  Discrete Derivative : simulink/Discrete/Discrete Derivative  gainval=1.0  ICPrevScaledInput=0.0  OutMin=[]  OutMax=[]  OutDataType=fixdt(1, 16)  OutScaling=2^-10  DoSatur=off
  Gain : Gain  Gain=1/(starshot.magnetorq.A*starshot.magnetorq.n)
  Gain10 : Gain  Gain=starshot.controller.Kp*starshot.IC.massproperties.Izp
  Gain11 : Gain  Gain=starshot.controller.Kd*starshot.IC.massproperties.Izp
  Mux1 : Mux  Inputs=3
  Mux2 : Mux  Inputs=3
  Norm2 : Subsystem
  Norm3 : Subsystem
  Product4 : Product  Multiplication=Matrix(*)
  Product6 : Product  Inputs=*/
  Product7 : Product  Inputs=**/
  Product8 : Product  Inputs=**
  Saturation3 : Saturate  UpperLimit=starshot.magnetorq.m_max_x/(starshot.magnetorq.A*starshot.magnetorq.n)  LowerLimit=-starshot.magnetorq.m_max_x/(starshot.magnetorq.A*starshot.magnetorq.n)
  Saturation4 : Saturate  UpperLimit=starshot.magnetorq.m_max_y/(starshot.magnetorq.A*starshot.magnetorq.n)  LowerLimit=-starshot.magnetorq.m_max_y/(starshot.magnetorq.A*starshot.magnetorq.n)
  Saturation5 : Saturate  UpperLimit=starshot.magnetorq.m_max_z/(starshot.magnetorq.A*starshot.magnetorq.n)  LowerLimit=-starshot.magnetorq.m_max_z/(starshot.magnetorq.A*starshot.magnetorq.n)
  Sign : Signum
  Skew matrix S(tau_c)1 : Subsystem
  Subsystem1 : Subsystem
  Sum7 : Sum  Inputs=+|+
  Trigonometric Function5 : Trigonometry  Operator=asin
  e_z : Constant  Value=[0 0 1]
  sign_function1 : Subsystem
  Dipole : Outport
  wires:
  Product4/1 -> Product6/1
  Mux2/1 -> Gain/1
  Sum7/1 -> Product7/2
  Trigonometric Function5/1 -> Gain10/1, Discrete Derivative/1
  Norm3/1(norm(v)) -> Trigonometric Function5/1
  e_z/1 -> Skew matrix S(tau_c)1/1(omega)
  Product7/1 -> Mux2/3
  Constant12/1 -> Mux2/2, Mux2/1
  Skew matrix S(tau_c)1/1(S(omega)) -> Product4/1
  Discrete Derivative/1 -> Gain11/1
  Norm2/1(norm(v)) -> Product7/3, Product6/2
  Gain10/1 -> Sum7/1
  Product6/1 -> Norm3/1(v)
  Product8/1 -> Product7/1
  Gain11/1 -> Sum7/2
  B(body)/1 -> Product4/2, Norm2/1(v), Subsystem1/2(B(body))
  Subsystem1/1(sign(cos)) -> Product8/2
  Omega/1 -> Demux/1, Subsystem1/1(omega)
  Gain/1 -> Demux12/1
  Demux12/1 -> Saturation3/1
  Saturation3/1 -> Mux1/1
  Saturation5/1 -> Mux1/3
  Demux12/2 -> Saturation4/1
  Saturation4/1 -> Mux1/2
  Demux12/3 -> Saturation5/1
  Mux1/1 -> Dipole/1
  Demux/3 -> Cos/1
  Cos/1 -> Sign/1
  Sign/1 -> Product8/1

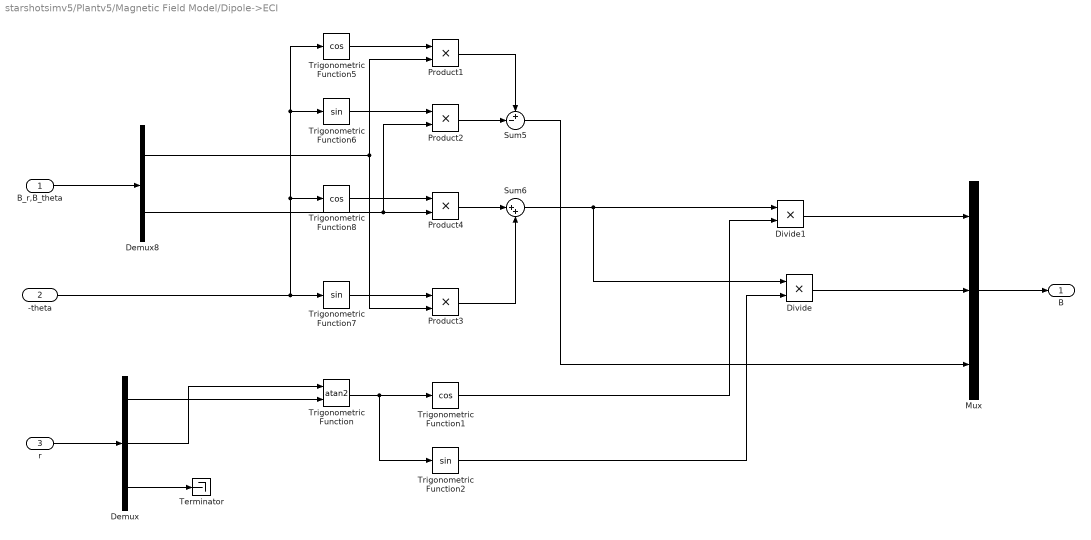
== system starshotsimv5/Plantv5/Magnetic Field Model/Dipole->ECI ==
  B_r,B_theta : Inport
  -theta : Inport  Port=2
  r : Inport  Port=3
  Demux : Demux  Outputs=3
  Demux8 : Demux  Outputs=2
  Divide : Product  Inputs=**
  Divide1 : Product  Inputs=**
  Mux : Mux  Inputs=3
  Product{1..4} (4 alike) : Product
  Sum5 : Sum  Inputs=+-|
  Sum6 : Sum  Inputs=|++
  Terminator : Terminator
  Trigonometric Function : Trigonometry  Operator=atan2
  Trigonometric Function1 : Trigonometry  Operator=cos
  Trigonometric Function2 : Trigonometry
  Trigonometric Function5 : Trigonometry  Operator=cos
  Trigonometric Function6 : Trigonometry
  Trigonometric Function7 : Trigonometry
  Trigonometric Function8 : Trigonometry  Operator=cos
  B : Outport
  wires:
  -theta/1 -> Trigonometric Function5/1, Trigonometric Function6/1, Trigonometric Function8/1, Trigonometric Function7/1
  Product4/1 -> Sum6/1
  Product3/1 -> Sum6/2
  Demux8/1 -> Product3/2, Product1/2
  Demux8/2 -> Product2/2, Product4/2
  Trigonometric Function5/1 -> Product1/1
  Product2/1 -> Sum5/2
  Trigonometric Function7/1 -> Product3/1
  B_r,B_theta/1 -> Demux8/1
  Sum5/1 -> Mux/3
  Trigonometric Function8/1 -> Product4/1
  Trigonometric Function6/1 -> Product2/1
  Sum6/1 -> Divide1/1, Divide/1
  Product1/1 -> Sum5/1
  r/1 -> Demux/1
  Demux/3 -> Terminator/1
  Demux/2 -> Trigonometric Function/1
  Demux/1 -> Trigonometric Function/2
  Trigonometric Function/1 -> Trigonometric Function1/1, Trigonometric Function2/1
  Trigonometric Function1/1 -> Divide1/2
  Trigonometric Function2/1 -> Divide/2
  Mux/1 -> B/1
  Divide1/1 -> Mux/1
  Divide/1 -> Mux/2

== system starshotsimv5/Plantv5/Quaternion Integration/q_normalize ==
  q_in : Inport  PortDimensions=4
  Dot Product : DotProduct  InputSameDT=on  OutDataTypeStr=Inherit: Inherit via internal rule
  Math Function : Math  Operator=sqrt  SignedPower=on  SaturateOnIntegerOverflow=on
  Product : Product  Inputs=*/  InputSameDT=on  SaturateOnIntegerOverflow=on  OutDataTypeStr=Inherit: Same as first input
  q_out : Outport
  wires:
  Product/1 -> q_out/1
  Math Function/1 -> Product/2
  Dot Product/1 -> Math Function/1
  q_in/1 -> Dot Product/2, Dot Product/1, Product/1

== system starshotsimv5/Plantv5/Quaternion Integration/qderiv ==
  w : Inport
  q : Inport  Port=2
  Mux : Mux  Inputs=2
  Mux1 : Mux
  qd1 : Fcn  Expr=(u(7)*u(1)-u(6)*u(2)+u(5)*u(3))/2
  qd2 : Fcn  Expr=(u(6)*u(1)+u(7)*u(2)-u(4)*u(3))/2
  qd3 : Fcn  Expr=(-u(5)*u(1)+u(4)*u(2)+u(7)*u(3))/2
  qd4 : Fcn  Expr=(-u(4)*u(1)-u(5)*u(2)-u(6)*u(3))/2
  qd : Outport
  wires:
  Mux1/1 -> qd/1
  qd4/1 -> Mux1/4
  qd3/1 -> Mux1/3
  qd2/1 -> Mux1/2
  qd1/1 -> Mux1/1
  Mux/1 -> qd4/1, qd3/1, qd2/1, qd1/1
  q/1 -> Mux/2
  w/1 -> Mux/1

== system starshotsimv5/Plantv5/qtoQ/Subsystem ==
  In1 : Inport
  3x3 : Reshape  OutputDimensionality=Customize  OutputDimensions=[3,3]
  Demux : Demux  Outputs=3
      settings: DisplayOption=none
  Gain : Gain  Gain=-1  SaturateOnIntegerOverflow=on  OutDataTypeStr=Inherit: Same as input  ParamDataTypeStr=Inherit: Same as input
  Gain1 : Gain  Gain=-1  SaturateOnIntegerOverflow=on  OutDataTypeStr=Inherit: Same as input  ParamDataTypeStr=Inherit: Same as input
  Gain2 : Gain  Gain=-1  SaturateOnIntegerOverflow=on  OutDataTypeStr=Inherit: Same as input  ParamDataTypeStr=Inherit: Same as input
  Mux : Mux  Inputs=9
  "diag 0 " : Constant  Value=0
  Out1 : Outport
  wires:
  Gain2/1 -> Mux/8
  Demux/1 -> Gain2/1, Mux/6
  Gain1/1 -> Mux/4
  Demux/2 -> Mux/7, Gain/1
  Gain/1 -> Mux/3
  Demux/3 -> Gain1/1, Mux/2
  Mux/1 -> 3x3/1
  "diag 0 "/1 -> Mux/9, Mux/5, Mux/1
  3x3/1 -> Out1/1
  In1/1 -> Demux/1

== system starshotsimv5/Plantv5/qtoQ1/Subsystem ==
  In1 : Inport
  3x3 : Reshape  OutputDimensionality=Customize  OutputDimensions=[3,3]
  Demux : Demux  Outputs=3
      settings: DisplayOption=none
  Gain : Gain  Gain=-1  SaturateOnIntegerOverflow=on  OutDataTypeStr=Inherit: Same as input  ParamDataTypeStr=Inherit: Same as input
  Gain1 : Gain  Gain=-1  SaturateOnIntegerOverflow=on  OutDataTypeStr=Inherit: Same as input  ParamDataTypeStr=Inherit: Same as input
  Gain2 : Gain  Gain=-1  SaturateOnIntegerOverflow=on  OutDataTypeStr=Inherit: Same as input  ParamDataTypeStr=Inherit: Same as input
  Mux : Mux  Inputs=9
  "diag 0 " : Constant  Value=0
  Out1 : Outport
  wires:
  In1/1 -> Demux/1
  3x3/1 -> Out1/1
  "diag 0 "/1 -> Mux/1, Mux/5, Mux/9
  Mux/1 -> 3x3/1
  Demux/3 -> Mux/2, Gain1/1
  Gain/1 -> Mux/3
  Demux/2 -> Gain/1, Mux/7
  Gain1/1 -> Mux/4
  Demux/1 -> Mux/6, Gain2/1
  Gain2/1 -> Mux/8

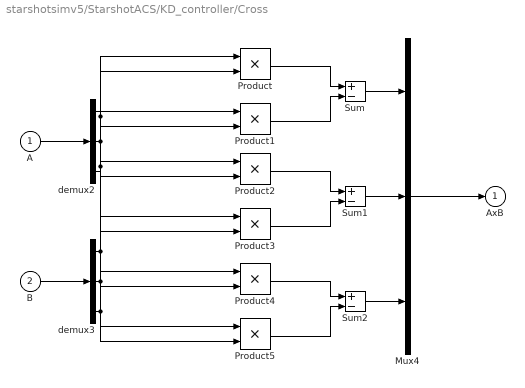
== system starshotsimv5/StarshotACS/KD_controller/Cross ==
  A : Inport
  B : Inport  Port=2
  Mux4 : Mux  Inputs=3
  Product{,1..5} (6 alike) : Product  InputSameDT=on  SaturateOnIntegerOverflow=on  OutDataTypeStr=Inherit: Same as first input
  Sum : Sum  Inputs=+-  InputSameDT=on  SaturateOnIntegerOverflow=on  OutDataTypeStr=Inherit: Same as first input
  Sum1 : Sum  Inputs=+-  InputSameDT=on  SaturateOnIntegerOverflow=on  OutDataTypeStr=Inherit: Same as first input
  Sum2 : Sum  Inputs=+-  InputSameDT=on  SaturateOnIntegerOverflow=on  OutDataTypeStr=Inherit: Same as first input
  demux2 : Demux  Outputs=3
      settings: DisplayOption=none
  demux3 : Demux  Outputs=3
      settings: DisplayOption=none
  AxB : Outport  InitialOutput=0
  wires:
  A/1 -> demux2/1
  B/1 -> demux3/1
  demux2/3 -> Product1/1, Product2/1
  demux3/3 -> Product/2, Product3/2
  demux2/1 -> Product3/1, Product4/1
  demux3/2 -> Product1/2, Product4/2
  demux2/2 -> Product/1, Product5/1
  demux3/1 -> Product2/2, Product5/2
  Product/1 -> Sum/1
  Product1/1 -> Sum/2
  Product2/1 -> Sum1/1
  Product3/1 -> Sum1/2
  Product4/1 -> Sum2/1
  Product5/1 -> Sum2/2
  Sum/1 -> Mux4/1
  Sum1/1 -> Mux4/2
  Sum2/1 -> Mux4/3
  Mux4/1 -> AxB/1

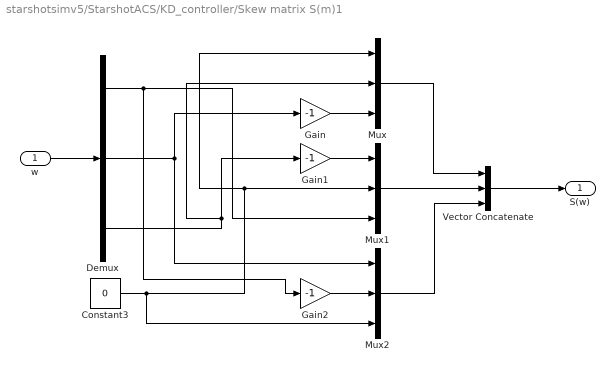
== system starshotsimv5/StarshotACS/KD_controller/Skew matrix S(m)1 ==
  w : Inport
  Constant3 : Constant  Value=0
  Demux : Demux  Outputs=3
  Gain : Gain  Gain=-1
  Gain1 : Gain  Gain=-1
  Gain2 : Gain  Gain=-1
  Mux : Mux  Inputs=3
  Mux1 : Mux  Inputs=3
  Mux2 : Mux  Inputs=3
  Vector Concatenate : Concatenate  NumInputs=3  Mode=Multidimensional array  ConcatenateDimension=2
  S(w) : Outport
  wires:
  Gain/1 -> Mux/3
  Demux/2 -> Mux2/1, Gain/1
  Demux/3 -> Gain1/1, Mux/2
  Gain2/1 -> Mux2/2
  Demux/1 -> Mux1/3, Gain2/1
  Mux1/1 -> Vector Concatenate/2
  w/1 -> Demux/1
  Constant3/1 -> Mux2/3, Mux/1, Mux1/2
  Vector Concatenate/1 -> S(w)/1
  Mux/1 -> Vector Concatenate/1
  Mux2/1 -> Vector Concatenate/3
  Gain1/1 -> Mux1/1

== system starshotsimv5/StarshotACS/Orientation controller/Norm2 ==
  v : Inport
  Dot Product6 : DotProduct  InputSameDT=on  OutDataTypeStr=Inherit: Inherit via internal rule
  Sqrt4 : Sqrt  SaturateOnIntegerOverflow=on
  norm(v) : Outport
  wires:
  v/1 -> Dot Product6/1, Dot Product6/2
  Dot Product6/1 -> Sqrt4/1
  Sqrt4/1 -> norm(v)/1

== system starshotsimv5/StarshotACS/Orientation controller/Norm3 ==
  v : Inport
  Dot Product6 : DotProduct  InputSameDT=on  OutDataTypeStr=Inherit: Inherit via internal rule
  Sqrt4 : Sqrt  SaturateOnIntegerOverflow=on
  norm(v) : Outport
  wires:
  v/1 -> Dot Product6/1, Dot Product6/2
  Dot Product6/1 -> Sqrt4/1
  Sqrt4/1 -> norm(v)/1

== system starshotsimv5/StarshotACS/Orientation controller/Skew matrix S(tau_c)1 ==
  omega : Inport
  Constant3 : Constant  Value=0
  Demux : Demux  Outputs=3
  Gain : Gain  Gain=-1
  Gain1 : Gain  Gain=-1
  Gain2 : Gain  Gain=-1
  Mux : Mux  Inputs=3
  Mux1 : Mux  Inputs=3
  Mux2 : Mux  Inputs=3
  Vector Concatenate : Concatenate  NumInputs=3  Mode=Multidimensional array  ConcatenateDimension=2
  S(omega) : Outport
  wires:
  Gain/1 -> Mux/3
  Demux/2 -> Mux2/1, Gain/1  "2"
  Demux/3 -> Gain1/1, Mux/2  "3"
  Gain2/1 -> Mux2/2
  Demux/1 -> Mux1/3, Gain2/1  "1"
  Mux1/1 -> Vector Concatenate/2
  omega/1 -> Demux/1
  Constant3/1 -> Mux2/3, Mux/1, Mux1/2  "0"
  Vector Concatenate/1 -> S(omega)/1
  Mux/1 -> Vector Concatenate/1
  Mux2/1 -> Vector Concatenate/3
  Gain1/1 -> Mux1/1

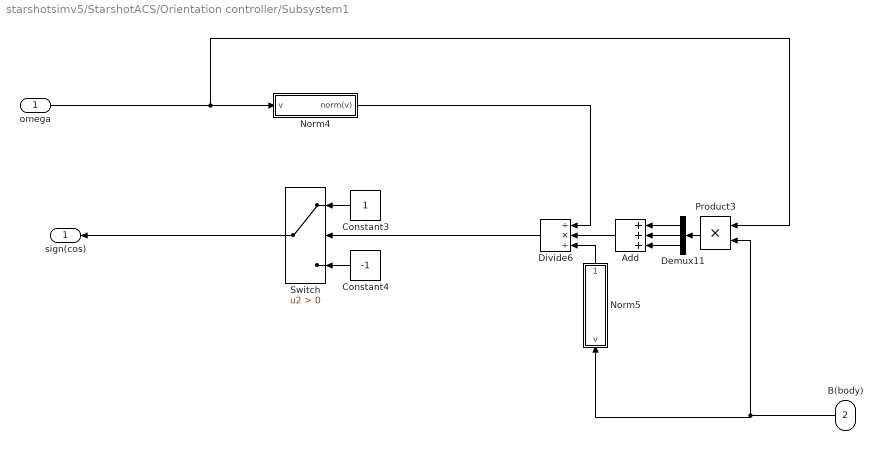
== system starshotsimv5/StarshotACS/Orientation controller/Subsystem1 ==
  omega : Inport
  B(body) : Inport  Port=2
  Add : Sum  Inputs=3
  Constant3 : Constant
  Constant4 : Constant  Value=-1
  Demux11 : Demux  Outputs=3
  Divide6 : Product  Inputs=/*/
  Norm4 : Subsystem
  Norm5 : Subsystem
  Product3 : Product
  Switch : Switch  Criteria=u2 > Threshold  ZeroCross=off
  sign(cos) : Outport
  wires:
  Switch/1 -> sign(cos)/1
  Constant4/1 -> Switch/3
  Add/1 -> Divide6/2
  Constant3/1 -> Switch/1
  Demux11/3 -> Add/3
  Norm4/1(norm(v)) -> Divide6/1
  Divide6/1 -> Switch/2
  Norm5/1(norm(v)) -> Divide6/3
  Product3/1 -> Demux11/1
  Demux11/1 -> Add/1
  Demux11/2 -> Add/2
  B(body)/1 -> Norm5/1(v), Product3/2
  omega/1 -> Product3/1, Norm4/1(v)

== system starshotsimv5/StarshotACS/Orientation controller/sign_function1 ==
  omega : Inport
  Constant10 : Constant  Value=-1
  Constant9 : Constant
  Selector : Selector  InputPortWidth=3  IndexOptions=Index vector (dialog)  Indices=[3]  OutputSizes=1
  Switch1 : Switch  ZeroCross=off
  sign(omega_z) : Outport
  wires:
  Constant9/1 -> Switch1/1
  Constant10/1 -> Switch1/3
  Switch1/1 -> sign(omega_z)/1
  Selector/1 -> Switch1/2
  omega/1 -> Selector/1

== system starshotsimv5/StarshotACS/Orientation controller/Subsystem1/Norm4 ==
  v : Inport
  Dot Product6 : DotProduct  InputSameDT=on  OutDataTypeStr=Inherit: Inherit via internal rule
  Sqrt4 : Sqrt  SaturateOnIntegerOverflow=on
  norm(v) : Outport
  wires:
  v/1 -> Dot Product6/1, Dot Product6/2
  Dot Product6/1 -> Sqrt4/1
  Sqrt4/1 -> norm(v)/1

== system starshotsimv5/StarshotACS/Orientation controller/Subsystem1/Norm5 ==
  v : Inport
  Dot Product6 : DotProduct  InputSameDT=on  OutDataTypeStr=Inherit: Inherit via internal rule
  Sqrt4 : Sqrt  SaturateOnIntegerOverflow=on
  norm(v) : Outport
  wires:
  v/1 -> Dot Product6/1, Dot Product6/2
  Dot Product6/1 -> Sqrt4/1
  Sqrt4/1 -> norm(v)/1

== matlab function starshotsimv5/EKF/EKF_Primary/Kalman corrector ==
  data: Z input; X_k1_k1 output; X_k1_k input; P_k1_k input; P_k1_k1 output; Hd parameter; Rd parameter
function [X_k1_k1, P_k1_k1] = fcn(Z, X_k1_k, P_k1_k, Hd, Rd)


initial = Z;
disp(initial);
K_k1 = P_k1_k * Hd' * inv(Hd*P_k1_k*Hd' + Rd);
P_k1_k1 = P_k1_k - K_k1*(Hd*P_k1_k*Hd' + Rd)*K_k1';
X_k1_k1 = X_k1_k + K_k1* (Z - Hd*X_k1_k);

== matlab function starshotsimv5/EKF/Jacobian ==
  data: B_body input; J output; angular_velocities input
function J = fcn(B_body, angular_velocities)

Bx = B_body(1);
By = B_body(2);
Bz = B_body(3);
wx = angular_velocities(1);
wy = angular_velocities(2);
wz = angular_velocities(3);

J = [ 0, wz, -wy, 0, -Bz, By; ...
    -wz, 0, wx, Bz, 0, -Bx; ...
     wy, - wx, 0, -By, Bx, 0; ...
     0, 0, 0, 0, -wz, -wy; ...
     0, 0, 0, wz, 0, wx; ...
     0, 0, 0, -wx/3, -wy/3, 0];

== matlab function starshotsimv5/EKF/EKF_Primary/Kalman predictor ==
  data: J_k_k input; X_k1_k output; X_k_k input; P_k_k input; P_k1_k output; dT parameter; Q parameter
function [X_k1_k, P_k1_k] = fcn(J_k_k, X_k_k, P_k_k, dT, Q)

delta_t = 0.1;
F = @(t,y)[-y(3)*y(5)+y(2)*y(6); y(3)*y(4)-y(1)*y(6); -y(2)*y(4)+y(1)*y(5);-y(5)*y(6);y(4)*y(6);-y(4)*y(5)/3];
tspan = (0:0.0001:delta_t);

y0 = X_k_k;

[~,sol] = ode45(F,tspan,y0);
%disp(sol(end,1:end));
%disp("One iter");

A = J_k_k;

Ad = expm(A*dT);

%disp(X_k_k);

X_k1_k = sol(end,1:end)'; 
P_k1_k = Ad*P_k_k*Ad' + Q;

== matlab function starshotsimv5/EKF/EKF_Primary/sqrt(Pii) ==
  data: u input; y output
function y = fcn(u)

y = norm(u);
disp(y);
